simulink model "linearization_pendulum_model"  (R2024b)
settings: Solver=ode3  StartTime=0.0  StopTime=t(end)  RelTol=1e-3
undefined symbols (not defined in the file): g, J_pend, J_rotor, kr, kt, R, U, uv_dc, uv_pend
settings Model: Creator=Student  LastModifiedBy=Paweł Wiktor
settings SolverCC: AlgebraicLoopSolver=TrustRegion
settings DataIOCC: ReturnWorkspaceOutputs=off
settings DebuggingCC: UnconnectedInputMsg=warning  UnconnectedOutputMsg=warning  UnconnectedLineMsg=warning  ArithmeticOperatorsInVariantConditions=warning
settings ModelReferenceCC: EnableRefExpFcnMdlSchedulingChecks=on
settings SFSimCC: CustomCodeUndefinedFunction=UseInterfaceOnly
settings RTWCC: GPUComputeCapability=3.5

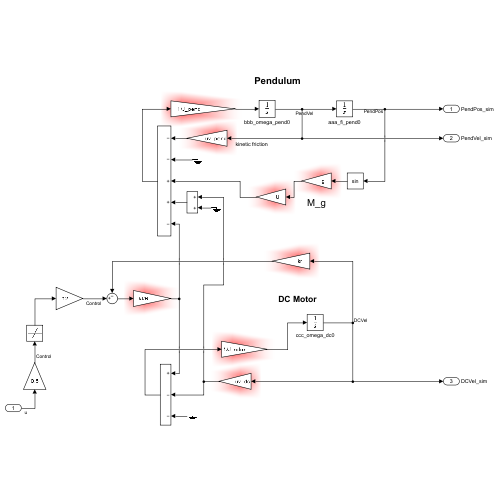
[thumbnail: Simulink's stored preview of the top-level diagram]
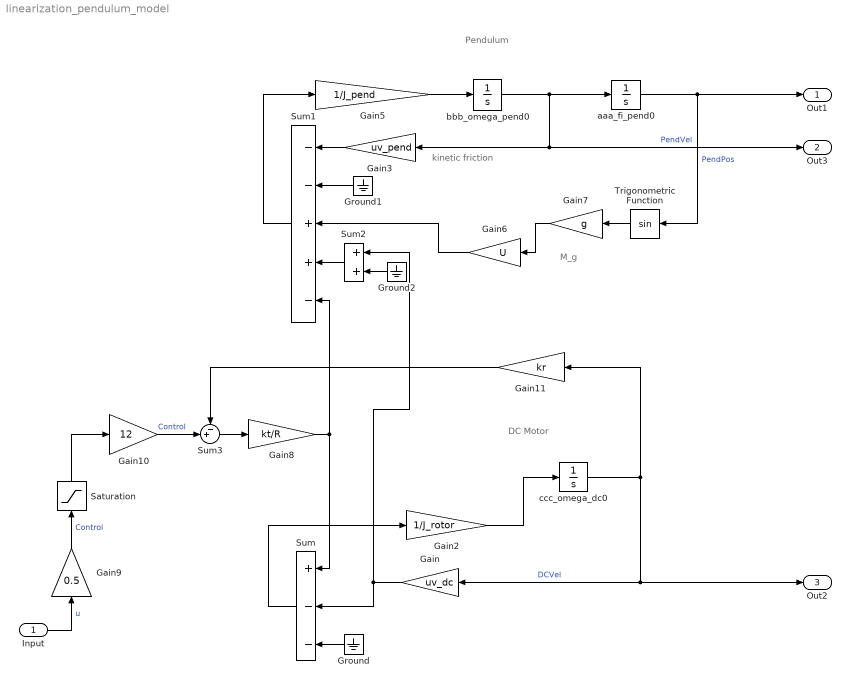
== system linearization_pendulum_model ==
  note: DC Motor
  note: Pendulum
  note: kinetic friction
  note: M_g
  Input : Inport
  Gain : Gain  Gain=uv_dc
  Gain10 : Gain  Gain=12
  Gain11 : Gain  Gain=kr
  Gain2 : Gain  Gain=1/J_rotor
  Gain3 : Gain  Gain=uv_pend
  Gain5 : Gain  Gain=1/J_pend
  Gain6 : Gain  Gain=U
  Gain7 : Gain  Gain=g
  Gain8 : Gain  Gain=kt/R
  Gain9 : Gain  Gain=0.5
  Ground : Ground
  Ground1 : Ground
  Ground2 : Ground
  Saturation : Saturate  UpperLimit=1  LowerLimit=-1
  Sum : Sum  Inputs=+--
  Sum1 : Sum  Inputs=--++-
  Sum2 : Sum
  Sum3 : Sum  Inputs=-+|
  Trigonometric Function : Trigonometry
  aaa_fi_pend0 : Integrator
  bbb_omega_pend0 : Integrator
  ccc_omega_dc0 : Integrator
  Out1 : Outport  SignalName=PendPos_sim  VectorParamsAs1DForOutWhenUnconnected=off
  Out3 : Outport  Port=2  SignalName=PendVel_sim  VectorParamsAs1DForOutWhenUnconnected=off
  Out2 : Outport  Port=3  SignalName=DCVel_sim  VectorParamsAs1DForOutWhenUnconnected=off
  wires:
  ccc_omega_dc0/1 -> Gain11/1, Out2/1, Gain/1  "DCVel"
  Gain2/1 -> ccc_omega_dc0/1
  Sum/1 -> Gain2/1
  Gain6/1 -> Sum1/3
  Input/1 -> Gain9/1  "u"
  Gain7/1 -> Gain6/1
  Sum1/1 -> Gain5/1
  bbb_omega_pend0/1 -> Out3/1, Gain3/1, aaa_fi_pend0/1  "PendVel"
  Gain3/1 -> Sum1/1
  Trigonometric Function/1 -> Gain7/1
  aaa_fi_pend0/1 -> Trigonometric Function/1, Out1/1  "PendPos"
  Gain5/1 -> bbb_omega_pend0/1
  Gain8/1 -> Sum1/5, Sum/1
  Gain/1 -> Sum/2, Sum2/1
  Sum2/1 -> Sum1/4
  Gain9/1 -> Saturation/1  "Control"
  Gain10/1 -> Sum3/2  "Control"
  Saturation/1 -> Gain10/1
  Sum3/1 -> Gain8/1
  Gain11/1 -> Sum3/1
  Ground/1 -> Sum/3
  Ground1/1 -> Sum1/2
  Ground2/1 -> Sum2/2
